simulink model "simulink1mass"  (R2015a)
settings: Solver=ode15s  StartTime=0.0  StopTime=y_final  RelTol=1e-3
values from neighbouring files (symbols this model uses):
  c1 = str2num(get(handles.c1t,'String'))    [guiproject.m]
  k1 = str2num(get(handles.k1t,'String'))    [guiproject.m]
  m1 = str2num(get(handles.m1t,'String'))    [guiproject.m]
  y_final = str2num(get(handles.y_finalt,'String'))    [guiproject.m]
settings Model: Creator=b00058261  LastModifiedBy=b00058261

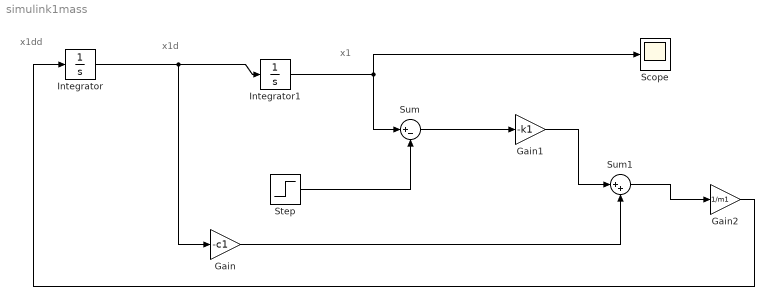
== system simulink1mass ==
  note: x1
  note: x1d
  note: x1dd
  Gain : Gain  Gain=-c1
  Gain1 : Gain  Gain=-k1
  Gain2 : Gain  Gain=1/m1
  Integrator : Integrator
  Integrator1 : Integrator
  Scope : Scope
      settings: SaveName=mass_1
  Step : Step  Time=0  After=y_final  SampleTime=0
  Sum : Sum  Inputs=|+-
  Sum1 : Sum  Inputs=|++
  wires:
  Integrator/1 -> Integrator1/1, Gain/1
  Integrator1/1 -> Scope/1, Sum/1
  Sum/1 -> Gain1/1
  Gain1/1 -> Sum1/1
  Gain/1 -> Sum1/2
  Sum1/1 -> Gain2/1
  Gain2/1 -> Integrator/1
  Step/1 -> Sum/2
